simulink model "simmodel"  (Simulink 9.0)
settings: Solver=ode1  StartTime=0.0  StopTime=5  FixedStep=0.0001  RelTol=1e-3
values from neighbouring files (symbols this model uses):
  A = [-a 0 -b ... (first row only)    [Initialize_Parameters.m]    (also in Initialize_Parameters_MATLAB_Functions.m)
  B = [c ... (first row only)    [Initialize_Parameters.m]    (also in Initialize_Parameters_MATLAB_Functions.m)
undefined symbols (not defined in the file or in its folder): Model_626, Sensoray
libraries: sldrtlib x4, simulink x1
settings Model: Creator=pawestlu  LastModifiedBy=lyericl
settings DataIOCC: SaveFormat=Dataset
settings OptimizationCC: LifeSpan=auto
settings DebuggingCC: UnderspecifiedInitializationDetection=Simplified  MergeDetectMultiDrivingBlocksExec=error  SFUnexpectedBacktrackingDiag=error  SFNoUnconditionalDefaultTransitionDiag=error  SFExecutionAtInitializationDiag=warning
settings HardwareCC: ProdBitPerPointer=64  ProdBitPerSizeT=64  ProdBitPerPtrDiffT=64  ProdLargestAtomicFloat=Float  ProdIntDivRoundTo=Zero  ProdEndianess=LittleEndian  ProdWordSize=64  ProdHWDeviceType=Intel->x86-64 (Windows64)
settings ModelReferenceCC: PropagateSignalLabelsOutOfModel=on
settings RTWCC: SystemTargetFile=sldrt.tlc  TemplateMakefile=sldrt.tmf  Description=Simulink Desktop Real-Time  RTWCompilerOptimization=on
settings CodeAppCC: MaxIdLength=95  StateflowObjectComments=off
settings SimulinkDesktopRealTimeCC: TargetPreCompLibLocation=C:\Program Files\MATLAB\R2017b\toolbox\sldrt\lib\win64
settings ConfigComp: CovMetricSettings=dwe  CovHtmlReporting=off  CovSaveCumulativeToWorkspaceVar=off  CovSaveSingleToWorkspaceVar=off  CovExternalEMLEnable=on

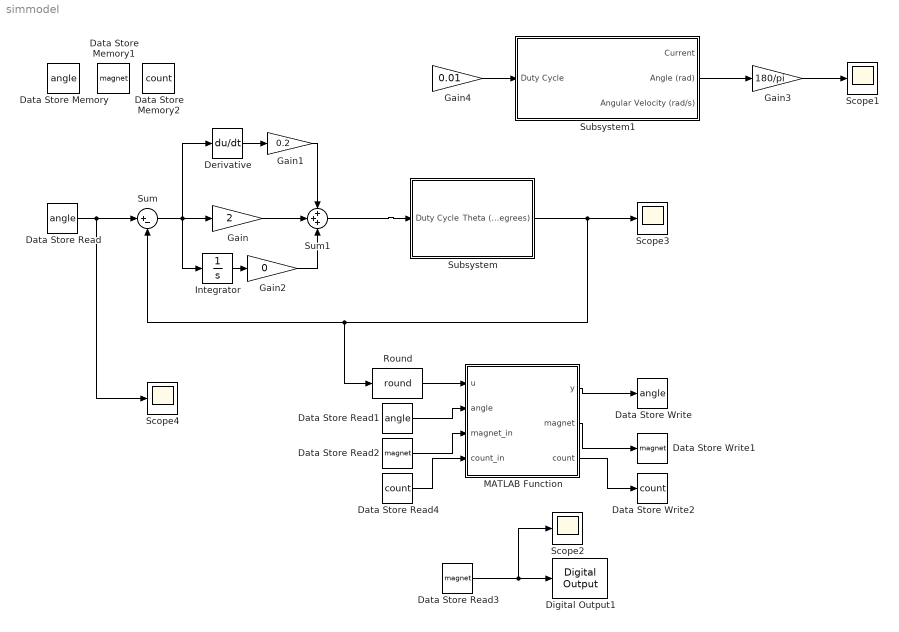
== system simmodel ==
  Data Store Memory : DataStoreMemory  DataStoreName=angle  ReadBeforeWriteMsg=warning  WriteAfterWriteMsg=warning  WriteAfterReadMsg=warning  InitialValue=90  ShowAdditionalParam=off
  Data Store Memory1 : DataStoreMemory  DataStoreName=magnet  ReadBeforeWriteMsg=warning  WriteAfterWriteMsg=warning  WriteAfterReadMsg=warning  InitialValue=5  ShowAdditionalParam=off
  Data Store Memory2 : DataStoreMemory  DataStoreName=count  ReadBeforeWriteMsg=warning  WriteAfterWriteMsg=warning  WriteAfterReadMsg=warning  ShowAdditionalParam=off
  Data Store Read : DataStoreRead  DataStoreName=angle
  Data Store Read1 : DataStoreRead  DataStoreName=angle
  Data Store Read2 : DataStoreRead  DataStoreName=magnet
  Data Store Read3 : DataStoreRead  DataStoreName=magnet
  Data Store Read4 : DataStoreRead  DataStoreName=count
  Data Store Write : DataStoreWrite  DataStoreName=angle
  Data Store Write1 : DataStoreWrite  DataStoreName=magnet
  Data Store Write2 : DataStoreWrite  DataStoreName=count
  Derivative : Derivative
  Digital Output1 : sldrtlib/Digital Output  SampleTime=0.0001  MaxMissedTicks=inf  ShowMissedTicks=off  YieldWhenWaiting=off  DrvName=Sensoray/Model_626  DrvAddress=4294967295  DrvOptions=zeros(1,0)  Channels=3  BitMode=1  InitialValue=5  FinalValue=5
      settings: AttributesFormatString=Sensoray\nModel 626 [auto]  SourceProductName=Simulink Desktop Real-Time  SourceProductBaseCode=WT
  Gain : Gain  Gain=2
  Gain1 : Gain  Gain=0.2
  Gain2 : Gain  Gain=0
  Gain3 : Gain  Gain=180/pi
  Gain4 : Gain  Gain=0.01
  Integrator : Integrator
  MATLAB Function : MATLAB Function  TreatAsAtomicUnit=on
  Round : Rounding  Operator=round
  Scope{1..4} (4 alike) : Scope
  Subsystem : Subsystem
  Subsystem1 : Subsystem
  Sum : Sum  Inputs=|+-
  Sum1 : Sum  Inputs=+++
  wires:
  Subsystem/1(Theta (degrees)) -> Scope3/1, Round/1, Sum/2
  Derivative/1 -> Gain1/1
  Gain1/1 -> Sum1/1
  Gain/1 -> Sum1/2
  Sum1/1 -> Subsystem/1(Duty Cycle)
  Integrator/1 -> Gain2/1
  Gain2/1 -> Sum1/3
  Subsystem1/2(Angle (rad)) -> Gain3/1
  Gain3/1 -> Scope1/1
  Gain4/1 -> Subsystem1/1(Duty Cycle)
  Sum/1 -> Derivative/1, Integrator/1, Gain/1
  Round/1 -> MATLAB Function/1(u)
  MATLAB Function/1(y) -> Data Store Write/1
  Data Store Read1/1 -> MATLAB Function/2(angle)
  Data Store Read/1 -> Scope4/1, Sum/1
  Data Store Read2/1 -> MATLAB Function/3(magnet_in)
  MATLAB Function/2(magnet) -> Data Store Write1/1
  Data Store Read3/1 -> Scope2/1, Digital Output1/1
  Data Store Read4/1 -> MATLAB Function/4(count_in)
  MATLAB Function/3(count) -> Data Store Write2/1

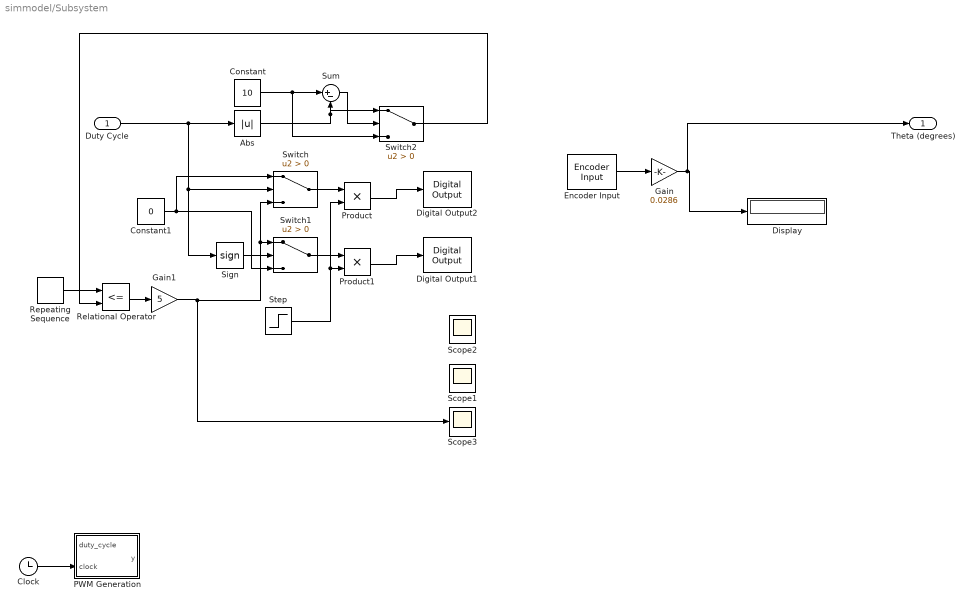
== system simmodel/Subsystem ==
  Duty Cycle : Inport
  Abs : Abs
  Clock : Clock
  Constant : Constant  Value=10  SampleTime=0.0001
  Constant1 : Constant  Value=0  SampleTime=0.0001
  Digital Output1 : sldrtlib/Digital Output  SampleTime=0.0001  MaxMissedTicks=inf  ShowMissedTicks=off  YieldWhenWaiting=off  DrvName=Sensoray/Model_626  DrvAddress=4294967295  DrvOptions=zeros(1,0)  Channels=2  BitMode=1  InitialValue=[]  FinalValue=[]
      settings: AttributesFormatString=Sensoray\nModel 626 [auto]  SourceProductName=Simulink Desktop Real-Time  SourceProductBaseCode=WT
  Digital Output2 : sldrtlib/Digital Output  SampleTime=0.0001  MaxMissedTicks=inf  ShowMissedTicks=off  YieldWhenWaiting=off  DrvName=Sensoray/Model_626  DrvAddress=4294967295  DrvOptions=zeros(1,0)  Channels=1  BitMode=1  InitialValue=[]  FinalValue=[]
      settings: AttributesFormatString=Sensoray\nModel 626 [auto]  SourceProductName=Simulink Desktop Real-Time  SourceProductBaseCode=WT
  Display : Display
  Encoder Input : sldrtlib/Encoder Input  SampleTime=0.0001  MaxMissedTicks=inf  ShowMissedTicks=off  YieldWhenWaiting=off  DrvName=Sensoray/Model_626  DrvAddress=4294967295  DrvOptions=zeros(1,0)  Channels=1  QuadMode=3  IndexPulse=2  InputFilter=Inf  DataType=1
      settings: AttributesFormatString=Sensoray\nModel 626 [auto]  SourceProductName=Simulink Desktop Real-Time
  Gain : Gain  Gain=0.0286
  Gain1 : Gain  Gain=5
  PWM Generation : MATLAB Function  TreatAsAtomicUnit=on
  Product : Product
  Product1 : Product
  Relational Operator : RelationalOperator  Operator=<=  OutDataTypeStr=boolean  RndMeth=Simplest
  Repeating Sequence : simulink/Sources/Repeating Sequence  rep_seq_t=[0 0.01]  rep_seq_y=[0 1]
  Scope1 : Scope
  Scope2 : Scope
  Scope3 : Scope
  Sign : Signum
  Step : Step  Time=4.9999  Before=1  After=0  SampleTime=0.0001
  Sum : Sum  Inputs=|+-
  Switch : Switch  Criteria=u2 > Threshold
  Switch1 : Switch  Criteria=u2 > Threshold
  Switch2 : Switch  Criteria=u2 > Threshold
  Theta (degrees) : Outport
  wires:
  Encoder Input/1 -> Gain/1
  Gain/1 -> Theta (degrees)/1, Display/1
  Duty Cycle/1 -> Sign/1, Switch/2, Abs/1
  Sign/1 -> Switch1/2
  Abs/1 -> Switch2/1, Sum/2
  Constant/1 -> Switch2/3, Sum/1
  Sum/1 -> Switch2/2
  Clock/1 -> PWM Generation/2(clock)
  Constant1/1 -> Switch1/3, Switch/1
  Switch1/1 -> Product1/1
  Switch/1 -> Product/1
  Product/1 -> Digital Output2/1
  Product1/1 -> Digital Output1/1
  Step/1 -> Product1/2, Product/2
  Repeating Sequence/1 -> Relational Operator/1
  Relational Operator/1 -> Gain1/1
  Switch2/1 -> Relational Operator/2
  Gain1/1 -> Switch/3, Switch1/1, Scope3/1

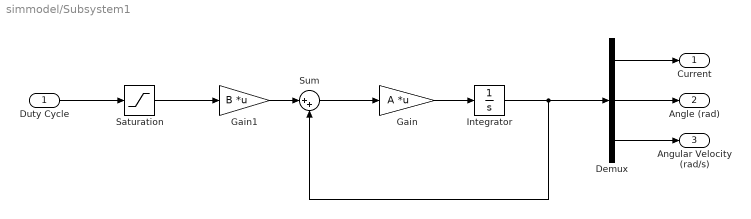
== system simmodel/Subsystem1 ==
  Duty Cycle : Inport
  Demux : Demux  Outputs=3
  Gain : Gain  Gain=A  Multiplication=Matrix(K*u)
  Gain1 : Gain  Gain=B  Multiplication=Matrix(K*u)
  Integrator : Integrator
  Saturation : Saturate  UpperLimit=1  LowerLimit=-1
  Sum : Sum  Inputs=|++
  Current : Outport
  Angle (rad) : Outport  Port=2
  Angular Velocity (rad/s) : Outport  Port=3
  wires:
  Sum/1 -> Gain/1
  Gain1/1 -> Sum/1
  Demux/2 -> Angle (rad)/1
  Gain/1 -> Integrator/1
  Integrator/1 -> Demux/1, Sum/2
  Duty Cycle/1 -> Saturation/1
  Demux/1 -> Current/1
  Demux/3 -> Angular Velocity (rad/s)/1
  Saturation/1 -> Gain1/1

== matlab function MATLAB Function ==
  data: u input double; y output double; angle input double; magnet output double; magnet_in input double; count_in input double; count output double
function [y, magnet, count] = fcn(u, angle, magnet_in, count_in)
if u == 90 && angle == 90
    if(count_in == 1)
        y = 45;
        magnet = 0;
        count = 0;
    else
        y = angle;
        magnet = 0;
        count = count_in + 1;
    end
    
else if u == 45 && angle == 45
    y = 45;
    if(count_in == 2000)
        magnet = 5;
        count = count_in;
    else
        magnet = magnet_in;
        count = count_in + 1;
    end
else
    y = angle;
    magnet = magnet_in;
    count = count_in;
    
end
end

== matlab function Subsystem/PWM Generation ==
  data: duty_cycle input double; y output double; clock input double
function y = fcn(duty_cycle, clock)
   
    amplitude_min = 0;
    amplitude_max = 5;
    period = 0.01;
    
    period_time = mod(clock, period) + 0.0001;
    
    if(period_time*100 <= duty_cycle)
        y = amplitude_max;
    else
        y = amplitude_min;
    end
end
